simulink model "PID_GA"  (R2025a)
settings: Solver=VariableStepAuto  StartTime=0.0  StopTime=20  RelTol=1e-3
undefined symbols (not defined in the file or in its folder): Kd1, Kd2, Ki1, Ki2, Kp1, Kp2
settings Model: Creator=nnajianthony  LastModifiedBy=edward

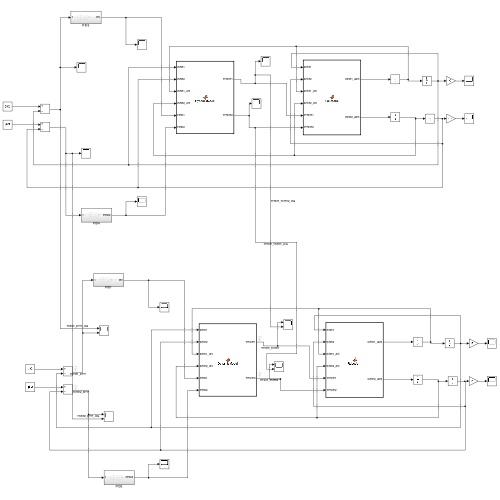
[thumbnail: Simulink's stored preview of the top-level diagram]
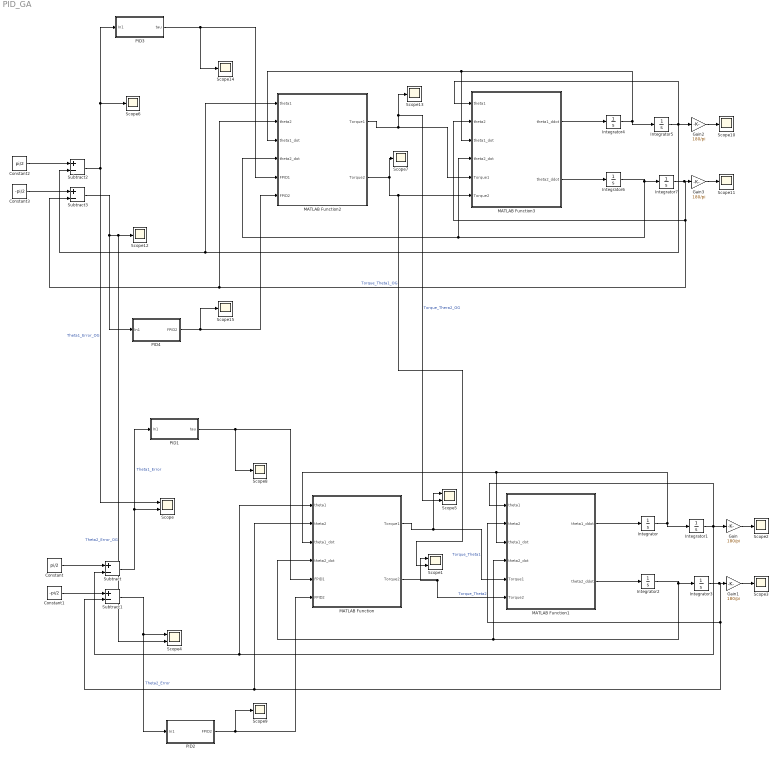
== system PID_GA ==
  Constant : Constant  Value=pi/2
  Constant1 : Constant  Value=-pi/2
  Constant2 : Constant  Value=pi/2
  Constant3 : Constant  Value=-pi/2
  Gain{,1..3} (4 alike) : Gain  Gain=180/pi
  Integrator{,2,4,6} (4 alike) : Integrator
  Integrator1 : Integrator  InitialCondition=-pi/2
  Integrator3 : Integrator  InitialCondition=pi/2
  Integrator5 : Integrator  InitialCondition=-pi/2
  Integrator7 : Integrator  InitialCondition=pi/2
  MATLAB Function : MATLAB Function  TreatAsAtomicUnit=on
  MATLAB Function1 : MATLAB Function  TreatAsAtomicUnit=on
  MATLAB Function2 : MATLAB Function  TreatAsAtomicUnit=on
  MATLAB Function3 : MATLAB Function  TreatAsAtomicUnit=on
  PID1 : Subsystem
  PID2 : Subsystem
  PID3 : Subsystem
  PID4 : Subsystem
  Scope{,1,4..5} (4 alike) : Scope  NumInputPorts=2
      Scope settings: ActiveDisplayYMinimum=-2.3554576105433944  ActiveDisplayYMaximum=6.4282410478541125  YLabel=Theta1 Error (rads)
      Scope1 settings: ActiveDisplayYMinimum=-73.941113638818692  ActiveDisplayYMaximum=45.096397435407667  YLabel=Theta2 Torque
      Scope4 settings: ActiveDisplayYMinimum=-4.6632762955398412  ActiveDisplayYMaximum=3.6909099400367533  YLabel=Theta2 Error (rads)  DataLoggingVariableName=ScopeData4
      Scope5 settings: ActiveDisplayYMinimum=-44.256962360165744  ActiveDisplayYMaximum=87.837195381900386  YLabel=Theta1 Torque  DataLoggingVariableName=ScopeData5
  Scope{2..3,6..15} (12 alike) : Scope
      Scope10 settings: ActiveDisplayYMinimum=-1  ActiveDisplayYMaximum=1  DataLoggingVariableName=ScopeData6
      Scope11 settings: ActiveDisplayYMinimum=-1  ActiveDisplayYMaximum=1  DataLoggingVariableName=ScopeData7
      Scope12 settings: ActiveDisplayYMinimum=-3.6207955941244974  ActiveDisplayYMaximum=1.1712338112225464  DataLoggingVariableName=ScopeData10
      Scope13 settings: ActiveDisplayYMinimum=-34.451733972908904  ActiveDisplayYMaximum=86.747725561094072  DataLoggingVariableName=ScopeData11
      Scope14 settings: ActiveDisplayYMinimum=-1  ActiveDisplayYMaximum=1  DataLoggingVariableName=ScopeData12
      Scope15 settings: ActiveDisplayYMinimum=-1  ActiveDisplayYMaximum=1  DataLoggingVariableName=ScopeData13
      Scope2 settings: ActiveDisplayYMinimum=-1  ActiveDisplayYMaximum=1  DataLoggingVariableName=ScopeData2
      Scope3 settings: ActiveDisplayYMinimum=-1  ActiveDisplayYMaximum=1  DataLoggingVariableName=ScopeData3
      Scope6 settings: ActiveDisplayYMinimum=-1  ActiveDisplayYMaximum=1  DataLoggingVariableName=ScopeData14
      Scope7 settings: ActiveDisplayYMinimum=-16.116304839749631  ActiveDisplayYMaximum=16.498719292835396  DataLoggingVariableName=ScopeData15
      Scope8 settings: ActiveDisplayYMinimum=-29.792624138240008  ActiveDisplayYMaximum=76.758270188722264  DataLoggingVariableName=ScopeData8
      Scope9 settings: ActiveDisplayYMinimum=-1  ActiveDisplayYMaximum=1  DataLoggingVariableName=ScopeData9
  Subtract{,1..3} (4 alike) : Sum  Inputs=+-
  wires:
  Subtract1/1 -> PID2/1(In1), Scope4/1  "Theta2_Error"
  Constant1/1 -> Subtract1/1
  Constant/1 -> Subtract/1
  Integrator/1 -> Integrator1/1, MATLAB Function1/3(theta1_dot), MATLAB Function/3(theta1_dot)
  MATLAB Function1/1(theta1_ddot) -> Integrator/1
  MATLAB Function1/2(theta2_ddot) -> Integrator2/1
  Integrator2/1 -> MATLAB Function/4(theta2_dot), MATLAB Function1/4(theta2_dot), Integrator3/1
  Integrator1/1 -> MATLAB Function1/1(theta1), MATLAB Function/1(theta1), Subtract/2, Gain/1
  Integrator3/1 -> MATLAB Function1/2(theta2), MATLAB Function/2(theta2), Subtract1/2, Gain1/1
  Gain/1 -> Scope2/1
  Gain1/1 -> Scope3/1
  MATLAB Function/2(Torque2) -> Scope1/1, MATLAB Function1/6(Torque2)  "Torque_Theta2"
  PID1/1(tau) -> Scope8/1, MATLAB Function/5(FPID1)
  Subtract/1 -> PID1/1(In1), Scope/2  "Theta1_Error"
  PID2/1(FPID2) -> Scope9/1, MATLAB Function/6(FPID2)
  MATLAB Function/1(Torque1) -> Scope5/1, MATLAB Function1/5(Torque1)  "Torque_Theta1"
  MATLAB Function3/2(theta2_ddot) -> Integrator6/1
  Subtract3/1 -> Scope4/2, Scope12/1, PID4/1(In1)  "Theta2_Error_OG"
  PID3/1(tau) -> Scope14/1, MATLAB Function2/5(FPID1)
  PID4/1(FPID2) -> Scope15/1, MATLAB Function2/6(FPID2)
  Gain2/1 -> Scope10/1
  Gain3/1 -> Scope11/1
  Integrator5/1 -> MATLAB Function3/1(theta1), MATLAB Function2/1(theta1), Subtract2/2, Gain2/1
  Subtract2/1 -> Scope/1, Scope6/1, PID3/1(In1)  "Theta1_Error_OG"
  Constant2/1 -> Subtract2/1
  Integrator7/1 -> MATLAB Function3/2(theta2), MATLAB Function2/2(theta2), Subtract3/2, Gain3/1
  Integrator4/1 -> Integrator5/1, MATLAB Function3/3(theta1_dot), MATLAB Function2/3(theta1_dot)
  Integrator6/1 -> MATLAB Function2/4(theta2_dot), MATLAB Function3/4(theta2_dot), Integrator7/1
  Constant3/1 -> Subtract3/1
  MATLAB Function3/1(theta1_ddot) -> Integrator4/1
  MATLAB Function2/2(Torque2) -> Scope7/1, Scope1/2, MATLAB Function3/6(Torque2)  "Torque_Theta1_OG"
  MATLAB Function2/1(Torque1) -> Scope5/2, Scope13/1, MATLAB Function3/5(Torque1)  "Torque_Thera2_OG"

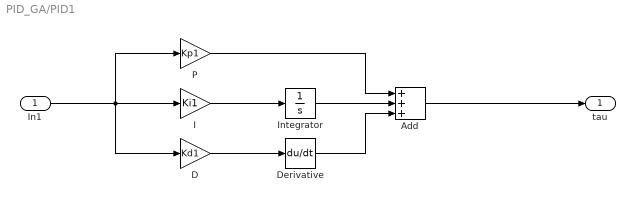
== system PID_GA/PID1 ==
  In1 : Inport
  Add : Sum  Inputs=+++
  D : Gain  Gain=Kd1
  Derivative : Derivative
  I : Gain  Gain=Ki1
  Integrator : Integrator
  P : Gain  Gain=Kp1
  tau : Outport
  wires:
  In1/1 -> D/1, P/1, I/1
  I/1 -> Integrator/1
  D/1 -> Derivative/1
  Add/1 -> tau/1
  Integrator/1 -> Add/2
  P/1 -> Add/1
  Derivative/1 -> Add/3

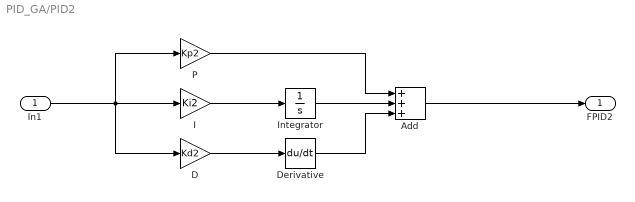
== system PID_GA/PID2 ==
  In1 : Inport
  Add : Sum  Inputs=+++
  D : Gain  Gain=Kd2
  Derivative : Derivative
  I : Gain  Gain=Ki2
  Integrator : Integrator
  P : Gain  Gain=Kp2
  FPID2 : Outport
  wires:
  Derivative/1 -> Add/3
  P/1 -> Add/1
  Integrator/1 -> Add/2
  Add/1 -> FPID2/1
  D/1 -> Derivative/1
  I/1 -> Integrator/1
  In1/1 -> I/1, P/1, D/1

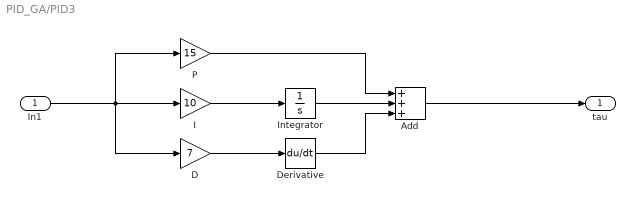
== system PID_GA/PID3 ==
  In1 : Inport
  Add : Sum  Inputs=+++
  D : Gain  Gain=7
  Derivative : Derivative
  I : Gain  Gain=10
  Integrator : Integrator
  P : Gain  Gain=15
  tau : Outport
  wires:
  In1/1 -> D/1, P/1, I/1
  I/1 -> Integrator/1
  D/1 -> Derivative/1
  Add/1 -> tau/1
  Integrator/1 -> Add/2
  P/1 -> Add/1
  Derivative/1 -> Add/3

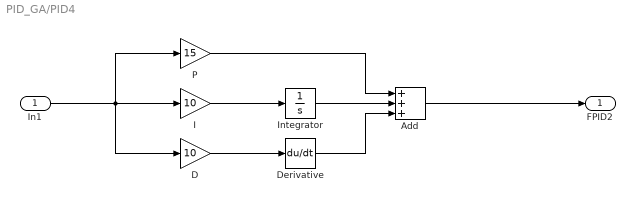
== system PID_GA/PID4 ==
  In1 : Inport
  Add : Sum  Inputs=+++
  D : Gain  Gain=10
  Derivative : Derivative
  I : Gain  Gain=10
  Integrator : Integrator
  P : Gain  Gain=15
  FPID2 : Outport
  wires:
  Derivative/1 -> Add/3
  P/1 -> Add/1
  Integrator/1 -> Add/2
  Add/1 -> FPID2/1
  D/1 -> Derivative/1
  I/1 -> Integrator/1
  In1/1 -> I/1, P/1, D/1

== matlab function PID_GA/MATLAB Function1 ==
  data: theta1 input; theta1_ddot output; theta2 input; theta1_dot input; theta2_dot input; Torque1 input; Torque2 input; theta2_ddot output
function [theta1_ddot, theta2_ddot] = RobotArm(theta1, theta2, theta1_dot, theta2_dot, Torque1, Torque2)
%#codegen

% Parameters
m1 = 1; m2 = 1;
l1 = 1; l2 = 1;
g = 9.81;

% Trig shortcuts
c2 = cos(theta2);
s2 = sin(theta2);
s1 = sin(theta1);
s12 = sin(theta1 + theta2);

%% Inertia Matrix M (from image)
D11 = (m1 + m2)*l1^2 + m2*l2^2 + 2*m2*l1*l2*c2;
D12 = m2*l2^2 + m2*l1*l2*c2;
D21 = D12;
D22 = m2*l2^2;
D = [D11, D12; D21, D22];

%% Coriolis and Centrifugal Vector C (from image)
C1 = -2*m2*l1*l2*s2*theta1_dot*theta2_dot - m2*l1*l2*s2*theta2_dot^2;
C2 = m2*l1*l2*s2*theta1_dot^2;
C = [C1; C2];

%% Gravity Vector G (from image)
G1 = (m1 + m2)*g*l1*s1 + m2*g*l2*s12;
G2 = m2*g*l2*s12;
G = [G1; G2];

% Compute acceleration
Tau = [Torque1; Torque2];
ddq = inv(D) * (Tau - C - G);

theta1_ddot = ddq(1);
theta2_ddot = ddq(2);
end

== matlab function PID_GA/MATLAB Function ==
  data: theta1 input; Torque1 output; theta2 input; theta1_dot input; theta2_dot input; FPID1 input; FPID2 input; Torque2 output
function [Torque1, Torque2] = DynamicModel(theta1, theta2, theta1_dot, theta2_dot, FPID1, FPID2)
%#codegen

% Parameters
m1 = 1; m2 = 1;
l1 = 1; l2 = 1;
g = 9.81;
% Trig shortcuts
c2 = cos(theta2);
s2 = sin(theta2);
s1 = sin(theta1);
s12 = sin(theta1 + theta2);

%% Inertia Matrix M (from image)
D11 = (m1 + m2)*l1^2 + m2*l2^2 + 2*m2*l1*l2*c2;
D12 = m2*l2^2 + m2*l1*l2*c2;
D21 = D12;
D22 = m2*l2^2;
D = [D11, D12; D21, D22];

%% Coriolis and Centrifugal Vector C (from image)
C1 = -2*m2*l1*l2*s2*theta1_dot*theta2_dot - m2*l1*l2*s2*theta2_dot^2;
C2 = m2*l1*l2*s2*theta1_dot^2;
C = [C1; C2];

%% Gravity Vector G (from image)
G1 = (m1 + m2)*g*l1*s1 + m2*g*l2*s12;
G2 = m2*g*l2*s12;
G = [G1; G2];

% Final torque
q_ddot = [FPID1; FPID2];
Torque = D * q_ddot + C + G;

Torque1 = Torque(1);
Torque2 = Torque(2);
end

== matlab function PID_GA/MATLAB Function2 ==
  data: theta1 input; Torque1 output; theta2 input; theta1_dot input; theta2_dot input; FPID1 input; FPID2 input; Torque2 output
function [Torque1, Torque2] = DynamicModel(theta1, theta2, theta1_dot, theta2_dot, FPID1, FPID2)
%#codegen

% Parameters
m1 = 1; m2 = 1;
l1 = 1; l2 = 1;
g = 9.81;
% Trig shortcuts
c2 = cos(theta2);
s2 = sin(theta2);
s1 = sin(theta1);
s12 = sin(theta1 + theta2);

%% Inertia Matrix M (from image)
D11 = (m1 + m2)*l1^2 + m2*l2^2 + 2*m2*l1*l2*c2;
D12 = m2*l2^2 + m2*l1*l2*c2;
D21 = D12;
D22 = m2*l2^2;
D = [D11, D12; D21, D22];

%% Coriolis and Centrifugal Vector C (from image)
C1 = -2*m2*l1*l2*s2*theta1_dot*theta2_dot - m2*l1*l2*s2*theta2_dot^2;
C2 = m2*l1*l2*s2*theta1_dot^2;
C = [C1; C2];

%% Gravity Vector G (from image)
G1 = (m1 + m2)*g*l1*s1 + m2*g*l2*s12;
G2 = m2*g*l2*s12;
G = [G1; G2];

% Final torque
q_ddot = [FPID1; FPID2];
Torque = D * q_ddot + C + G;

Torque1 = Torque(1);
Torque2 = Torque(2);
end

== matlab function PID_GA/MATLAB Function3 ==
  data: theta1 input; theta1_ddot output; theta2 input; theta1_dot input; theta2_dot input; Torque1 input; Torque2 input; theta2_ddot output
function [theta1_ddot, theta2_ddot] = RobotArm(theta1, theta2, theta1_dot, theta2_dot, Torque1, Torque2)
%#codegen

% Parameters
m1 = 1; m2 = 1;
l1 = 1; l2 = 1;
g = 9.81;

% Trig shortcuts
c2 = cos(theta2);
s2 = sin(theta2);
s1 = sin(theta1);
s12 = sin(theta1 + theta2);

%% Inertia Matrix M (from image)
D11 = (m1 + m2)*l1^2 + m2*l2^2 + 2*m2*l1*l2*c2;
D12 = m2*l2^2 + m2*l1*l2*c2;
D21 = D12;
D22 = m2*l2^2;
D = [D11, D12; D21, D22];

%% Coriolis and Centrifugal Vector C (from image)
C1 = -2*m2*l1*l2*s2*theta1_dot*theta2_dot - m2*l1*l2*s2*theta2_dot^2;
C2 = m2*l1*l2*s2*theta1_dot^2;
C = [C1; C2];

%% Gravity Vector G (from image)
G1 = (m1 + m2)*g*l1*s1 + m2*g*l2*s12;
G2 = m2*g*l2*s12;
G = [G1; G2];

% Compute acceleration
Tau = [Torque1; Torque2];
ddq = inv(D) * (Tau - C - G);

theta1_ddot = ddq(1);
theta2_ddot = ddq(2);
end
